simulink model "final_heart_sym3_5_Level_double"  (R2021a)
settings: Solver=VariableStepAuto  StartTime=0.0  StopTime=8  RelTol=1e-3
undefined symbols (not defined in the file): lambda2
libraries: dspsigops x11, dspquant2 x1
(part 3 of 3)

== system final_heart_sym3_5_Level_double/Threshold_Estimator/Median2/Data_Sorter11 ==
  Signal1 : Inport  OutDataTypeStr=double  SampleTime=1/44100
  Signal2 : Inport  Port=2  OutDataTypeStr=double  SampleTime=1/44100
  Data_Sorter_Switch : Switch  OutDataTypeStr=double
  Data_Sorter_Switch1 : Switch  Threshold=1  OutDataTypeStr=double
  Delay1 : Delay  DelayLength=1  SampleTime=1/44100
  Delay2 : Delay  DelayLength=1  SampleTime=1/44100
  Relational Operator2 : RelationalOperator  Operator=<  OutDataTypeStr=boolean  RndMeth=Simplest
  High_Data : Outport  OutDataTypeStr=double  SampleTime=1/44100  VectorParamsAs1DForOutWhenUnconnected=off
  Low_Data : Outport  Port=2  OutDataTypeStr=double  SampleTime=1/44100  VectorParamsAs1DForOutWhenUnconnected=off
  wires:
  Signal1/1 -> Data_Sorter_Switch/3, Data_Sorter_Switch/1, Relational Operator2/1
  Relational Operator2/1 -> Data_Sorter_Switch1/2, Data_Sorter_Switch/2
  Signal2/1 -> Data_Sorter_Switch1/1, Data_Sorter_Switch1/3, Relational Operator2/2
  Data_Sorter_Switch1/1 -> Delay2/1
  Delay2/1 -> Low_Data/1
  Data_Sorter_Switch/1 -> Delay1/1
  Delay1/1 -> High_Data/1

== system final_heart_sym3_5_Level_double/Threshold_Estimator/Median2/Data_Sorter12 ==
  Signal1 : Inport  OutDataTypeStr=double  SampleTime=1/44100
  Signal2 : Inport  Port=2  OutDataTypeStr=double  SampleTime=1/44100
  Data_Sorter_Switch : Switch  OutDataTypeStr=double
  Data_Sorter_Switch1 : Switch  Threshold=1  OutDataTypeStr=double
  Delay1 : Delay  DelayLength=1  SampleTime=1/44100
  Delay2 : Delay  DelayLength=1  SampleTime=1/44100
  Relational Operator2 : RelationalOperator  Operator=<  OutDataTypeStr=boolean  RndMeth=Simplest
  High_Data : Outport  OutDataTypeStr=double  SampleTime=1/44100  VectorParamsAs1DForOutWhenUnconnected=off
  Low_Data : Outport  Port=2  OutDataTypeStr=double  SampleTime=1/44100  VectorParamsAs1DForOutWhenUnconnected=off
  wires:
  Signal1/1 -> Data_Sorter_Switch/3, Data_Sorter_Switch/1, Relational Operator2/1
  Relational Operator2/1 -> Data_Sorter_Switch1/2, Data_Sorter_Switch/2
  Signal2/1 -> Data_Sorter_Switch1/1, Data_Sorter_Switch1/3, Relational Operator2/2
  Data_Sorter_Switch1/1 -> Delay2/1
  Delay2/1 -> Low_Data/1
  Data_Sorter_Switch/1 -> Delay1/1
  Delay1/1 -> High_Data/1

== system final_heart_sym3_5_Level_double/Threshold_Estimator/Median2/Data_Sorter13 ==
  Signal1 : Inport  OutDataTypeStr=double  SampleTime=1/44100
  Signal2 : Inport  Port=2  OutDataTypeStr=double  SampleTime=1/44100
  Data_Sorter_Switch : Switch  OutDataTypeStr=double
  Data_Sorter_Switch1 : Switch  Threshold=1  OutDataTypeStr=double
  Delay1 : Delay  DelayLength=1  SampleTime=1/44100
  Delay2 : Delay  DelayLength=1  SampleTime=1/44100
  Relational Operator2 : RelationalOperator  Operator=<  OutDataTypeStr=boolean  RndMeth=Simplest
  High_Data : Outport  OutDataTypeStr=double  SampleTime=1/44100  VectorParamsAs1DForOutWhenUnconnected=off
  Low_Data : Outport  Port=2  OutDataTypeStr=double  SampleTime=1/44100  VectorParamsAs1DForOutWhenUnconnected=off
  wires:
  Signal1/1 -> Data_Sorter_Switch/3, Data_Sorter_Switch/1, Relational Operator2/1
  Relational Operator2/1 -> Data_Sorter_Switch1/2, Data_Sorter_Switch/2
  Signal2/1 -> Data_Sorter_Switch1/1, Data_Sorter_Switch1/3, Relational Operator2/2
  Data_Sorter_Switch1/1 -> Delay2/1
  Delay2/1 -> Low_Data/1
  Data_Sorter_Switch/1 -> Delay1/1
  Delay1/1 -> High_Data/1

== system final_heart_sym3_5_Level_double/Threshold_Estimator/Median2/Data_Sorter14 ==
  Signal1 : Inport  OutDataTypeStr=double  SampleTime=1/44100
  Signal2 : Inport  Port=2  OutDataTypeStr=double  SampleTime=1/44100
  Data_Sorter_Switch : Switch  OutDataTypeStr=double
  Data_Sorter_Switch1 : Switch  Threshold=1  OutDataTypeStr=double
  Delay1 : Delay  DelayLength=1  SampleTime=1/44100
  Delay2 : Delay  DelayLength=1  SampleTime=1/44100
  Relational Operator2 : RelationalOperator  Operator=<  OutDataTypeStr=boolean  RndMeth=Simplest
  High_Data : Outport  OutDataTypeStr=double  SampleTime=1/44100  VectorParamsAs1DForOutWhenUnconnected=off
  Low_Data : Outport  Port=2  OutDataTypeStr=double  SampleTime=1/44100  VectorParamsAs1DForOutWhenUnconnected=off
  wires:
  Signal1/1 -> Data_Sorter_Switch/3, Data_Sorter_Switch/1, Relational Operator2/1
  Relational Operator2/1 -> Data_Sorter_Switch1/2, Data_Sorter_Switch/2
  Signal2/1 -> Data_Sorter_Switch1/1, Data_Sorter_Switch1/3, Relational Operator2/2
  Data_Sorter_Switch1/1 -> Delay2/1
  Delay2/1 -> Low_Data/1
  Data_Sorter_Switch/1 -> Delay1/1
  Delay1/1 -> High_Data/1

== system final_heart_sym3_5_Level_double/Threshold_Estimator/Median2/Data_Sorter15 ==
  Signal1 : Inport  OutDataTypeStr=double  SampleTime=1/44100
  Signal2 : Inport  Port=2  OutDataTypeStr=double  SampleTime=1/44100
  Data_Sorter_Switch1 : Switch  Threshold=1  OutDataTypeStr=double
  Delay2 : Delay  DelayLength=1  SampleTime=1/44100
  Relational Operator2 : RelationalOperator  Operator=<  OutDataTypeStr=boolean  RndMeth=Simplest
  Low_Data : Outport  OutDataTypeStr=double  SampleTime=1/44100  VectorParamsAs1DForOutWhenUnconnected=off
  wires:
  Signal1/1 -> Relational Operator2/1
  Relational Operator2/1 -> Data_Sorter_Switch1/2
  Signal2/1 -> Data_Sorter_Switch1/1, Data_Sorter_Switch1/3, Relational Operator2/2
  Data_Sorter_Switch1/1 -> Delay2/1
  Delay2/1 -> Low_Data/1

== system final_heart_sym3_5_Level_double/Threshold_Estimator/Median2/Data_Sorter16 ==
  Signal1 : Inport  OutDataTypeStr=double  SampleTime=1/44100
  Signal2 : Inport  Port=2  OutDataTypeStr=double  SampleTime=1/44100
  Data_Sorter_Switch : Switch  OutDataTypeStr=double
  Data_Sorter_Switch1 : Switch  Threshold=1  OutDataTypeStr=double
  Delay1 : Delay  DelayLength=1  SampleTime=1/44100
  Delay2 : Delay  DelayLength=1  SampleTime=1/44100
  Relational Operator2 : RelationalOperator  Operator=<  OutDataTypeStr=boolean  RndMeth=Simplest
  High_Data : Outport  OutDataTypeStr=double  SampleTime=1/44100  VectorParamsAs1DForOutWhenUnconnected=off
  Low_Data : Outport  Port=2  OutDataTypeStr=double  SampleTime=1/44100  VectorParamsAs1DForOutWhenUnconnected=off
  wires:
  Signal1/1 -> Data_Sorter_Switch/3, Data_Sorter_Switch/1, Relational Operator2/1
  Relational Operator2/1 -> Data_Sorter_Switch1/2, Data_Sorter_Switch/2
  Signal2/1 -> Data_Sorter_Switch1/1, Data_Sorter_Switch1/3, Relational Operator2/2
  Data_Sorter_Switch1/1 -> Delay2/1
  Delay2/1 -> Low_Data/1
  Data_Sorter_Switch/1 -> Delay1/1
  Delay1/1 -> High_Data/1

== system final_heart_sym3_5_Level_double/Threshold_Estimator/Median2/Data_Sorter17 ==
  Signal1 : Inport  OutDataTypeStr=double  SampleTime=1/44100
  Signal2 : Inport  Port=2  OutDataTypeStr=double  SampleTime=1/44100
  Data_Sorter_Switch : Switch  OutDataTypeStr=double
  Data_Sorter_Switch1 : Switch  Threshold=1  OutDataTypeStr=double
  Delay1 : Delay  DelayLength=1  SampleTime=1/44100
  Delay2 : Delay  DelayLength=1  SampleTime=1/44100
  Relational Operator2 : RelationalOperator  Operator=<  OutDataTypeStr=boolean  RndMeth=Simplest
  High_Data : Outport  OutDataTypeStr=double  SampleTime=1/44100  VectorParamsAs1DForOutWhenUnconnected=off
  Low_Data : Outport  Port=2  OutDataTypeStr=double  SampleTime=1/44100  VectorParamsAs1DForOutWhenUnconnected=off
  wires:
  Signal1/1 -> Data_Sorter_Switch/3, Data_Sorter_Switch/1, Relational Operator2/1
  Relational Operator2/1 -> Data_Sorter_Switch1/2, Data_Sorter_Switch/2
  Signal2/1 -> Data_Sorter_Switch1/1, Data_Sorter_Switch1/3, Relational Operator2/2
  Data_Sorter_Switch1/1 -> Delay2/1
  Delay2/1 -> Low_Data/1
  Data_Sorter_Switch/1 -> Delay1/1
  Delay1/1 -> High_Data/1

== system final_heart_sym3_5_Level_double/Threshold_Estimator/Median2/Data_Sorter18 ==
  Signal1 : Inport  OutDataTypeStr=double  SampleTime=1/44100
  Signal2 : Inport  Port=2  OutDataTypeStr=double  SampleTime=1/44100
  Data_Sorter_Switch : Switch  OutDataTypeStr=double
  Delay1 : Delay  DelayLength=1  SampleTime=1/44100
  Relational Operator2 : RelationalOperator  Operator=<  OutDataTypeStr=boolean  RndMeth=Simplest
  High_Data : Outport  OutDataTypeStr=double  SampleTime=1/44100  VectorParamsAs1DForOutWhenUnconnected=off
  wires:
  Signal1/1 -> Data_Sorter_Switch/3, Data_Sorter_Switch/1, Relational Operator2/1
  Relational Operator2/1 -> Data_Sorter_Switch/2
  Signal2/1 -> Relational Operator2/2
  Data_Sorter_Switch/1 -> Delay1/1
  Delay1/1 -> High_Data/1

== system final_heart_sym3_5_Level_double/Threshold_Estimator/Median2/Data_Sorter19 ==
  Signal1 : Inport  OutDataTypeStr=double  SampleTime=1/44100
  Signal2 : Inport  Port=2  OutDataTypeStr=double  SampleTime=1/44100
  Data_Sorter_Switch1 : Switch  Threshold=1  OutDataTypeStr=double
  Delay2 : Delay  DelayLength=1  SampleTime=1/44100
  Relational Operator2 : RelationalOperator  Operator=<  OutDataTypeStr=boolean  RndMeth=Simplest
  Low_Data : Outport  OutDataTypeStr=double  SampleTime=1/44100  VectorParamsAs1DForOutWhenUnconnected=off
  wires:
  Signal1/1 -> Relational Operator2/1
  Relational Operator2/1 -> Data_Sorter_Switch1/2
  Signal2/1 -> Data_Sorter_Switch1/1, Data_Sorter_Switch1/3, Relational Operator2/2
  Data_Sorter_Switch1/1 -> Delay2/1
  Delay2/1 -> Low_Data/1

== system final_heart_sym3_5_Level_double/Threshold_Estimator/Median2/Data_Sorter2 ==
  Signal1 : Inport  OutDataTypeStr=double  SampleTime=1/44100
  Signal2 : Inport  Port=2  OutDataTypeStr=double  SampleTime=1/44100
  Data_Sorter_Switch : Switch  OutDataTypeStr=double
  Data_Sorter_Switch1 : Switch  Threshold=1  OutDataTypeStr=double
  Delay1 : Delay  DelayLength=1  SampleTime=1/44100
  Delay2 : Delay  DelayLength=1  SampleTime=1/44100
  Relational Operator2 : RelationalOperator  Operator=<  OutDataTypeStr=boolean  RndMeth=Simplest
  High_Data : Outport  OutDataTypeStr=double  SampleTime=1/44100  VectorParamsAs1DForOutWhenUnconnected=off
  Low_Data : Outport  Port=2  OutDataTypeStr=double  SampleTime=1/44100  VectorParamsAs1DForOutWhenUnconnected=off
  wires:
  Signal1/1 -> Data_Sorter_Switch/3, Data_Sorter_Switch/1, Relational Operator2/1
  Relational Operator2/1 -> Data_Sorter_Switch1/2, Data_Sorter_Switch/2
  Signal2/1 -> Data_Sorter_Switch1/1, Data_Sorter_Switch1/3, Relational Operator2/2
  Data_Sorter_Switch1/1 -> Delay2/1
  Delay2/1 -> Low_Data/1
  Data_Sorter_Switch/1 -> Delay1/1
  Delay1/1 -> High_Data/1

== system final_heart_sym3_5_Level_double/Threshold_Estimator/Median2/Data_Sorter20 ==
  Signal1 : Inport  OutDataTypeStr=double  SampleTime=1/44100
  Signal2 : Inport  Port=2  OutDataTypeStr=double  SampleTime=1/44100
  Data_Sorter_Switch : Switch  OutDataTypeStr=double
  Data_Sorter_Switch1 : Switch  Threshold=1  OutDataTypeStr=double
  Delay1 : Delay  DelayLength=1  SampleTime=1/44100
  Delay2 : Delay  DelayLength=1  SampleTime=1/44100
  Relational Operator2 : RelationalOperator  Operator=<  OutDataTypeStr=boolean  RndMeth=Simplest
  High_Data : Outport  OutDataTypeStr=double  SampleTime=1/44100  VectorParamsAs1DForOutWhenUnconnected=off
  Low_Data : Outport  Port=2  OutDataTypeStr=double  SampleTime=1/44100  VectorParamsAs1DForOutWhenUnconnected=off
  wires:
  Signal1/1 -> Data_Sorter_Switch/3, Data_Sorter_Switch/1, Relational Operator2/1
  Relational Operator2/1 -> Data_Sorter_Switch1/2, Data_Sorter_Switch/2
  Signal2/1 -> Data_Sorter_Switch1/1, Data_Sorter_Switch1/3, Relational Operator2/2
  Data_Sorter_Switch1/1 -> Delay2/1
  Delay2/1 -> Low_Data/1
  Data_Sorter_Switch/1 -> Delay1/1
  Delay1/1 -> High_Data/1

== system final_heart_sym3_5_Level_double/Threshold_Estimator/Median2/Data_Sorter21 ==
  Signal1 : Inport  OutDataTypeStr=double  SampleTime=1/44100
  Signal2 : Inport  Port=2  OutDataTypeStr=double  SampleTime=1/44100
  Data_Sorter_Switch : Switch  OutDataTypeStr=double
  Delay1 : Delay  DelayLength=1  SampleTime=1/44100
  Relational Operator2 : RelationalOperator  Operator=<  OutDataTypeStr=boolean  RndMeth=Simplest
  High_Data : Outport  OutDataTypeStr=double  SampleTime=1/44100  VectorParamsAs1DForOutWhenUnconnected=off
  wires:
  Signal1/1 -> Data_Sorter_Switch/3, Data_Sorter_Switch/1, Relational Operator2/1
  Relational Operator2/1 -> Data_Sorter_Switch/2
  Signal2/1 -> Relational Operator2/2
  Data_Sorter_Switch/1 -> Delay1/1
  Delay1/1 -> High_Data/1

== system final_heart_sym3_5_Level_double/Threshold_Estimator/Median2/Data_Sorter22 ==
  Signal1 : Inport  OutDataTypeStr=double  SampleTime=1/44100
  Signal2 : Inport  Port=2  OutDataTypeStr=double  SampleTime=1/44100
  Data_Sorter_Switch1 : Switch  Threshold=1  OutDataTypeStr=double
  Delay2 : Delay  DelayLength=1  SampleTime=1/44100
  Relational Operator2 : RelationalOperator  Operator=<  OutDataTypeStr=boolean  RndMeth=Simplest
  Low_Data : Outport  OutDataTypeStr=double  SampleTime=1/44100  VectorParamsAs1DForOutWhenUnconnected=off
  wires:
  Signal1/1 -> Relational Operator2/1
  Relational Operator2/1 -> Data_Sorter_Switch1/2
  Signal2/1 -> Data_Sorter_Switch1/1, Data_Sorter_Switch1/3, Relational Operator2/2
  Data_Sorter_Switch1/1 -> Delay2/1
  Delay2/1 -> Low_Data/1

== system final_heart_sym3_5_Level_double/Threshold_Estimator/Median2/Data_Sorter23 ==
  Signal1 : Inport  OutDataTypeStr=double  SampleTime=1/44100
  Signal2 : Inport  Port=2  OutDataTypeStr=double  SampleTime=1/44100
  Data_Sorter_Switch : Switch  OutDataTypeStr=double
  Delay1 : Delay  DelayLength=1  SampleTime=1/44100
  Relational Operator2 : RelationalOperator  Operator=<  OutDataTypeStr=boolean  RndMeth=Simplest
  High_Data : Outport  OutDataTypeStr=double  SampleTime=1/44100  VectorParamsAs1DForOutWhenUnconnected=off
  wires:
  Signal1/1 -> Data_Sorter_Switch/3, Data_Sorter_Switch/1, Relational Operator2/1
  Relational Operator2/1 -> Data_Sorter_Switch/2
  Signal2/1 -> Relational Operator2/2
  Data_Sorter_Switch/1 -> Delay1/1
  Delay1/1 -> High_Data/1

== system final_heart_sym3_5_Level_double/Threshold_Estimator/Median2/Data_Sorter24 ==
  Signal1 : Inport  OutDataTypeStr=double  SampleTime=1/44100
  Signal2 : Inport  Port=2  OutDataTypeStr=double  SampleTime=1/44100
  Data_Sorter_Switch : Switch  OutDataTypeStr=double
  Data_Sorter_Switch1 : Switch  Threshold=1  OutDataTypeStr=double
  Delay1 : Delay  DelayLength=1  SampleTime=1/44100
  Delay2 : Delay  DelayLength=1  SampleTime=1/44100
  Relational Operator2 : RelationalOperator  Operator=<  OutDataTypeStr=boolean  RndMeth=Simplest
  High_Data : Outport  OutDataTypeStr=double  SampleTime=1/44100  VectorParamsAs1DForOutWhenUnconnected=off
  Low_Data : Outport  Port=2  OutDataTypeStr=double  SampleTime=1/44100  VectorParamsAs1DForOutWhenUnconnected=off
  wires:
  Signal1/1 -> Data_Sorter_Switch/3, Data_Sorter_Switch/1, Relational Operator2/1
  Relational Operator2/1 -> Data_Sorter_Switch1/2, Data_Sorter_Switch/2
  Signal2/1 -> Data_Sorter_Switch1/1, Data_Sorter_Switch1/3, Relational Operator2/2
  Data_Sorter_Switch1/1 -> Delay2/1
  Delay2/1 -> Low_Data/1
  Data_Sorter_Switch/1 -> Delay1/1
  Delay1/1 -> High_Data/1

== system final_heart_sym3_5_Level_double/Threshold_Estimator/Median2/Data_Sorter3 ==
  Signal1 : Inport  OutDataTypeStr=double  SampleTime=1/44100
  Signal2 : Inport  Port=2  OutDataTypeStr=double  SampleTime=1/44100
  Data_Sorter_Switch : Switch  OutDataTypeStr=double
  Data_Sorter_Switch1 : Switch  Threshold=1  OutDataTypeStr=double
  Delay1 : Delay  DelayLength=1  SampleTime=1/44100
  Delay2 : Delay  DelayLength=1  SampleTime=1/44100
  Relational Operator2 : RelationalOperator  Operator=<  OutDataTypeStr=boolean  RndMeth=Simplest
  High_Data : Outport  OutDataTypeStr=double  SampleTime=1/44100  VectorParamsAs1DForOutWhenUnconnected=off
  Low_Data : Outport  Port=2  OutDataTypeStr=double  SampleTime=1/44100  VectorParamsAs1DForOutWhenUnconnected=off
  wires:
  Signal1/1 -> Data_Sorter_Switch/3, Data_Sorter_Switch/1, Relational Operator2/1
  Relational Operator2/1 -> Data_Sorter_Switch1/2, Data_Sorter_Switch/2
  Signal2/1 -> Data_Sorter_Switch1/1, Data_Sorter_Switch1/3, Relational Operator2/2
  Data_Sorter_Switch1/1 -> Delay2/1
  Delay2/1 -> Low_Data/1
  Data_Sorter_Switch/1 -> Delay1/1
  Delay1/1 -> High_Data/1

== system final_heart_sym3_5_Level_double/Threshold_Estimator/Median2/Data_Sorter4 ==
  Signal1 : Inport  OutDataTypeStr=double  SampleTime=1/44100
  Signal2 : Inport  Port=2  OutDataTypeStr=double  SampleTime=1/44100
  Data_Sorter_Switch : Switch  OutDataTypeStr=double
  Data_Sorter_Switch1 : Switch  Threshold=1  OutDataTypeStr=double
  Delay1 : Delay  DelayLength=1  SampleTime=1/44100
  Delay2 : Delay  DelayLength=1  SampleTime=1/44100
  Relational Operator2 : RelationalOperator  Operator=<  OutDataTypeStr=boolean  RndMeth=Simplest
  High_Data : Outport  OutDataTypeStr=double  SampleTime=1/44100  VectorParamsAs1DForOutWhenUnconnected=off
  Low_Data : Outport  Port=2  OutDataTypeStr=double  SampleTime=1/44100  VectorParamsAs1DForOutWhenUnconnected=off
  wires:
  Signal1/1 -> Data_Sorter_Switch/3, Data_Sorter_Switch/1, Relational Operator2/1
  Relational Operator2/1 -> Data_Sorter_Switch1/2, Data_Sorter_Switch/2
  Signal2/1 -> Data_Sorter_Switch1/1, Data_Sorter_Switch1/3, Relational Operator2/2
  Data_Sorter_Switch1/1 -> Delay2/1
  Delay2/1 -> Low_Data/1
  Data_Sorter_Switch/1 -> Delay1/1
  Delay1/1 -> High_Data/1

== system final_heart_sym3_5_Level_double/Threshold_Estimator/Median2/Data_Sorter5 ==
  Signal1 : Inport  OutDataTypeStr=double  SampleTime=1/44100
  Signal2 : Inport  Port=2  OutDataTypeStr=double  SampleTime=1/44100
  Data_Sorter_Switch : Switch  OutDataTypeStr=double
  Data_Sorter_Switch1 : Switch  Threshold=1  OutDataTypeStr=double
  Delay1 : Delay  DelayLength=1  SampleTime=1/44100
  Delay2 : Delay  DelayLength=1  SampleTime=1/44100
  Relational Operator2 : RelationalOperator  Operator=<  OutDataTypeStr=boolean  RndMeth=Simplest
  High_Data : Outport  OutDataTypeStr=double  SampleTime=1/44100  VectorParamsAs1DForOutWhenUnconnected=off
  Low_Data : Outport  Port=2  OutDataTypeStr=double  SampleTime=1/44100  VectorParamsAs1DForOutWhenUnconnected=off
  wires:
  Signal1/1 -> Data_Sorter_Switch/3, Data_Sorter_Switch/1, Relational Operator2/1
  Relational Operator2/1 -> Data_Sorter_Switch1/2, Data_Sorter_Switch/2
  Signal2/1 -> Data_Sorter_Switch1/1, Data_Sorter_Switch1/3, Relational Operator2/2
  Data_Sorter_Switch1/1 -> Delay2/1
  Delay2/1 -> Low_Data/1
  Data_Sorter_Switch/1 -> Delay1/1
  Delay1/1 -> High_Data/1

== system final_heart_sym3_5_Level_double/Threshold_Estimator/Median2/Data_Sorter6 ==
  Signal1 : Inport  OutDataTypeStr=double  SampleTime=1/44100
  Signal2 : Inport  Port=2  OutDataTypeStr=double  SampleTime=1/44100
  Data_Sorter_Switch : Switch  OutDataTypeStr=double
  Data_Sorter_Switch1 : Switch  Threshold=1  OutDataTypeStr=double
  Delay1 : Delay  DelayLength=1  SampleTime=1/44100
  Delay2 : Delay  DelayLength=1  SampleTime=1/44100
  Relational Operator2 : RelationalOperator  Operator=<  OutDataTypeStr=boolean  RndMeth=Simplest
  High_Data : Outport  OutDataTypeStr=double  SampleTime=1/44100  VectorParamsAs1DForOutWhenUnconnected=off
  Low_Data : Outport  Port=2  OutDataTypeStr=double  SampleTime=1/44100  VectorParamsAs1DForOutWhenUnconnected=off
  wires:
  Signal1/1 -> Data_Sorter_Switch/3, Data_Sorter_Switch/1, Relational Operator2/1
  Relational Operator2/1 -> Data_Sorter_Switch1/2, Data_Sorter_Switch/2
  Signal2/1 -> Data_Sorter_Switch1/1, Data_Sorter_Switch1/3, Relational Operator2/2
  Data_Sorter_Switch1/1 -> Delay2/1
  Delay2/1 -> Low_Data/1
  Data_Sorter_Switch/1 -> Delay1/1
  Delay1/1 -> High_Data/1

== system final_heart_sym3_5_Level_double/Threshold_Estimator/Median2/Data_Sorter7 ==
  Signal1 : Inport  OutDataTypeStr=double  SampleTime=1/44100
  Signal2 : Inport  Port=2  OutDataTypeStr=double  SampleTime=1/44100
  Data_Sorter_Switch : Switch  OutDataTypeStr=double
  Data_Sorter_Switch1 : Switch  Threshold=1  OutDataTypeStr=double
  Delay1 : Delay  DelayLength=1  SampleTime=1/44100
  Delay2 : Delay  DelayLength=1  SampleTime=1/44100
  Relational Operator2 : RelationalOperator  Operator=<  OutDataTypeStr=boolean  RndMeth=Simplest
  High_Data : Outport  OutDataTypeStr=double  SampleTime=1/44100  VectorParamsAs1DForOutWhenUnconnected=off
  Low_Data : Outport  Port=2  OutDataTypeStr=double  SampleTime=1/44100  VectorParamsAs1DForOutWhenUnconnected=off
  wires:
  Signal1/1 -> Data_Sorter_Switch/3, Data_Sorter_Switch/1, Relational Operator2/1
  Relational Operator2/1 -> Data_Sorter_Switch1/2, Data_Sorter_Switch/2
  Signal2/1 -> Data_Sorter_Switch1/1, Data_Sorter_Switch1/3, Relational Operator2/2
  Data_Sorter_Switch1/1 -> Delay2/1
  Delay2/1 -> Low_Data/1
  Data_Sorter_Switch/1 -> Delay1/1
  Delay1/1 -> High_Data/1

== system final_heart_sym3_5_Level_double/Threshold_Estimator/Median2/Data_Sorter8 ==
  Signal1 : Inport  OutDataTypeStr=double  SampleTime=1/44100
  Signal2 : Inport  Port=2  OutDataTypeStr=double  SampleTime=1/44100
  Data_Sorter_Switch : Switch  OutDataTypeStr=double
  Data_Sorter_Switch1 : Switch  Threshold=1  OutDataTypeStr=double
  Delay1 : Delay  DelayLength=1  SampleTime=1/44100
  Delay2 : Delay  DelayLength=1  SampleTime=1/44100
  Relational Operator2 : RelationalOperator  Operator=<  OutDataTypeStr=boolean  RndMeth=Simplest
  High_Data : Outport  OutDataTypeStr=double  SampleTime=1/44100  VectorParamsAs1DForOutWhenUnconnected=off
  Low_Data : Outport  Port=2  OutDataTypeStr=double  SampleTime=1/44100  VectorParamsAs1DForOutWhenUnconnected=off
  wires:
  Signal1/1 -> Data_Sorter_Switch/3, Data_Sorter_Switch/1, Relational Operator2/1
  Relational Operator2/1 -> Data_Sorter_Switch1/2, Data_Sorter_Switch/2
  Signal2/1 -> Data_Sorter_Switch1/1, Data_Sorter_Switch1/3, Relational Operator2/2
  Data_Sorter_Switch1/1 -> Delay2/1
  Delay2/1 -> Low_Data/1
  Data_Sorter_Switch/1 -> Delay1/1
  Delay1/1 -> High_Data/1

== system final_heart_sym3_5_Level_double/Threshold_Estimator/Median2/Data_Sorter9 ==
  Signal1 : Inport  OutDataTypeStr=double  SampleTime=1/44100
  Signal2 : Inport  Port=2  OutDataTypeStr=double  SampleTime=1/44100
  Data_Sorter_Switch : Switch  OutDataTypeStr=double
  Data_Sorter_Switch1 : Switch  Threshold=1  OutDataTypeStr=double
  Delay1 : Delay  DelayLength=1  SampleTime=1/44100
  Delay2 : Delay  DelayLength=1  SampleTime=1/44100
  Relational Operator2 : RelationalOperator  Operator=<  OutDataTypeStr=boolean  RndMeth=Simplest
  High_Data : Outport  OutDataTypeStr=double  SampleTime=1/44100  VectorParamsAs1DForOutWhenUnconnected=off
  Low_Data : Outport  Port=2  OutDataTypeStr=double  SampleTime=1/44100  VectorParamsAs1DForOutWhenUnconnected=off
  wires:
  Signal1/1 -> Data_Sorter_Switch/3, Data_Sorter_Switch/1, Relational Operator2/1
  Relational Operator2/1 -> Data_Sorter_Switch1/2, Data_Sorter_Switch/2
  Signal2/1 -> Data_Sorter_Switch1/1, Data_Sorter_Switch1/3, Relational Operator2/2
  Data_Sorter_Switch1/1 -> Delay2/1
  Delay2/1 -> Low_Data/1
  Data_Sorter_Switch/1 -> Delay1/1
  Delay1/1 -> High_Data/1
